simulink model "arduino"  (R2022a)
settings: Solver=VariableStepAuto  StartTime=0.0  StopTime=10.0  RelTol=1e-3
values from neighbouring files (symbols this model uses):
  R_L = 287    [ac_init.m]
libraries: eeGeneralControl x5, simulink x3, slpidlib x2, aerolibatmos2 x1
settings Model: Creator=vzink  LastModifiedBy=vzink

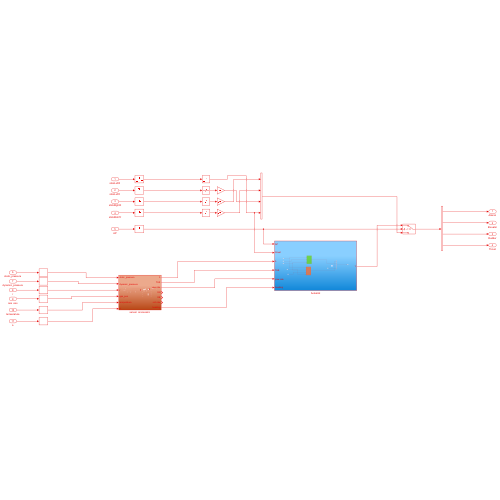
[thumbnail: Simulink's stored preview of the top-level diagram]
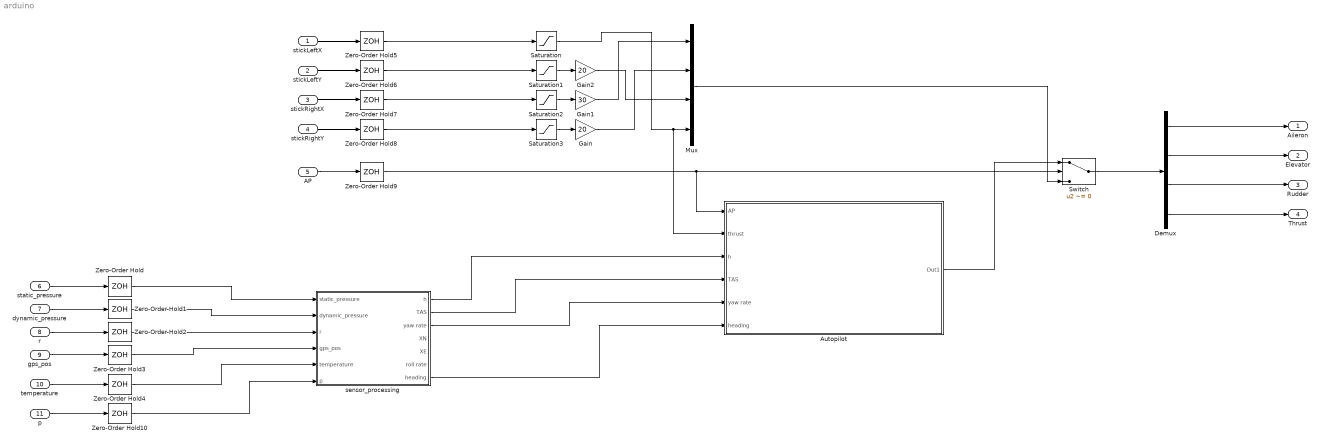
== system arduino ==
  stickLeftX : Inport
  stickLeftY : Inport  Port=2
  stickRightX : Inport  Port=3
  stickRightY : Inport  Port=4
  AP : Inport  Port=5
  static_pressure : Inport  Port=6
  dynamic_pressure : Inport  Port=7
  r : Inport  Port=8
  gps_pos : Inport  Port=9
  temperature : Inport  Port=10
  p : Inport  Port=11
  Autopilot : Subsystem
  Demux : Demux
  Gain : Gain  Gain=20
  Gain1 : Gain  Gain=30
  Gain2 : Gain  Gain=20
  Mux : Mux
  Saturation{,1..3} (4 alike) : Saturate  UpperLimit=1  LowerLimit=-1
  Switch : Switch  Criteria=u2 ~= 0  SaturateOnIntegerOverflow=off  InputSameDT=off
  Zero-Order Hold{,1..10} (11 alike) : ZeroOrderHold  SampleTime=0.01
  sensor_processing : Subsystem
  Aileron : Outport
  Elevator : Outport  Port=2
  Rudder : Outport  Port=3
  Thrust : Outport  Port=4
  wires:
  stickLeftX/1 -> Zero-Order Hold5/1
  stickLeftY/1 -> Zero-Order Hold6/1
  stickRightX/1 -> Zero-Order Hold7/1
  stickRightY/1 -> Zero-Order Hold8/1
  Saturation1/1 -> Gain2/1
  Saturation2/1 -> Gain1/1
  Saturation3/1 -> Gain/1
  Gain2/1 -> Mux/3
  Gain1/1 -> Mux/1
  Gain/1 -> Mux/2
  Saturation/1 -> Autopilot/2(thrust), Mux/4
  Mux/1 -> Switch/3
  Demux/1 -> Aileron/1
  Demux/2 -> Elevator/1
  Demux/3 -> Rudder/1
  Demux/4 -> Thrust/1
  Switch/1 -> Demux/1
  AP/1 -> Zero-Order Hold9/1
  static_pressure/1 -> Zero-Order Hold/1
  dynamic_pressure/1 -> Zero-Order Hold1/1
  r/1 -> Zero-Order Hold2/1
  gps_pos/1 -> Zero-Order Hold3/1
  temperature/1 -> Zero-Order Hold4/1
  sensor_processing/1(h) -> Autopilot/3(h)
  sensor_processing/2(TAS) -> Autopilot/4(TAS)
  sensor_processing/3(yaw rate) -> Autopilot/5(yaw rate)
  Zero-Order Hold/1 -> sensor_processing/1(static_pressure)
  Zero-Order Hold1/1 -> sensor_processing/2(dynamic_pressure)
  Zero-Order Hold2/1 -> sensor_processing/3(r)
  Zero-Order Hold3/1 -> sensor_processing/4(gps_pos)
  Zero-Order Hold4/1 -> sensor_processing/5(temperature)
  Zero-Order Hold5/1 -> Saturation/1
  Zero-Order Hold6/1 -> Saturation1/1
  Zero-Order Hold7/1 -> Saturation2/1
  Zero-Order Hold8/1 -> Saturation3/1
  Zero-Order Hold9/1 -> Autopilot/1(AP), Switch/2
  p/1 -> Zero-Order Hold10/1
  Zero-Order Hold10/1 -> sensor_processing/6(p)
  Autopilot/1(Out1) -> Switch/1
  sensor_processing/7(heading) -> Autopilot/6(heading)

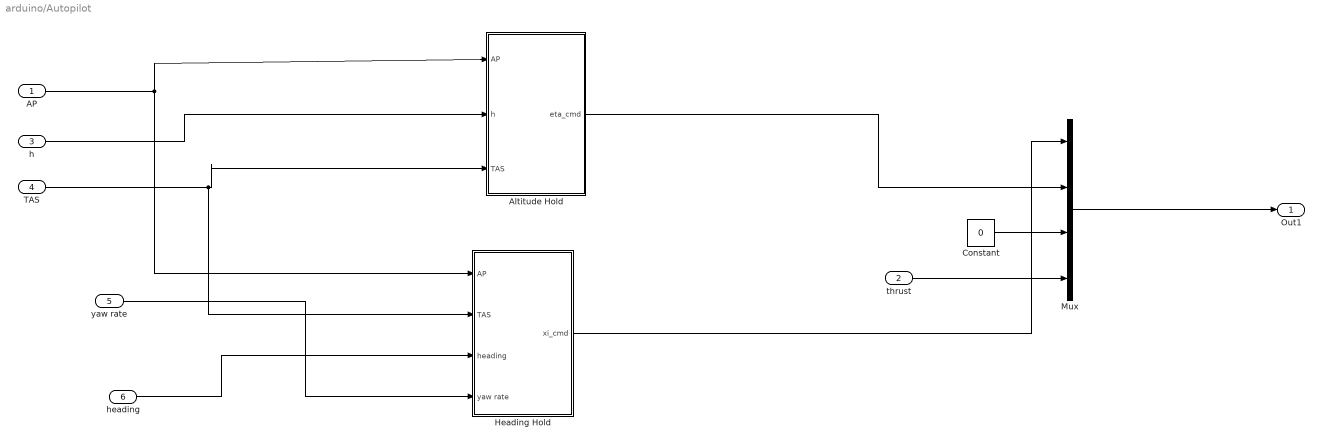
== system arduino/Autopilot ==
  AP : Inport
  thrust : Inport  Port=2
  h : Inport  Port=3
  TAS : Inport  Port=4
  yaw rate : Inport  Port=5
  heading : Inport  Port=6
  Altitude Hold : Subsystem
  Constant : Constant  Value=0
  Heading Hold : Subsystem
  Mux : Mux
  Out1 : Outport
  wires:
  Mux/1 -> Out1/1
  AP/1 -> Altitude Hold/1(AP), Heading Hold/1(AP)
  h/1 -> Altitude Hold/2(h)
  TAS/1 -> Heading Hold/2(TAS), Altitude Hold/3(TAS)
  Altitude Hold/1(eta_cmd) -> Mux/2
  thrust/1 -> Mux/4
  Constant/1 -> Mux/3
  Heading Hold/1(xi_cmd) -> Mux/1
  yaw rate/1 -> Heading Hold/4(yaw rate)
  heading/1 -> Heading Hold/3(heading)

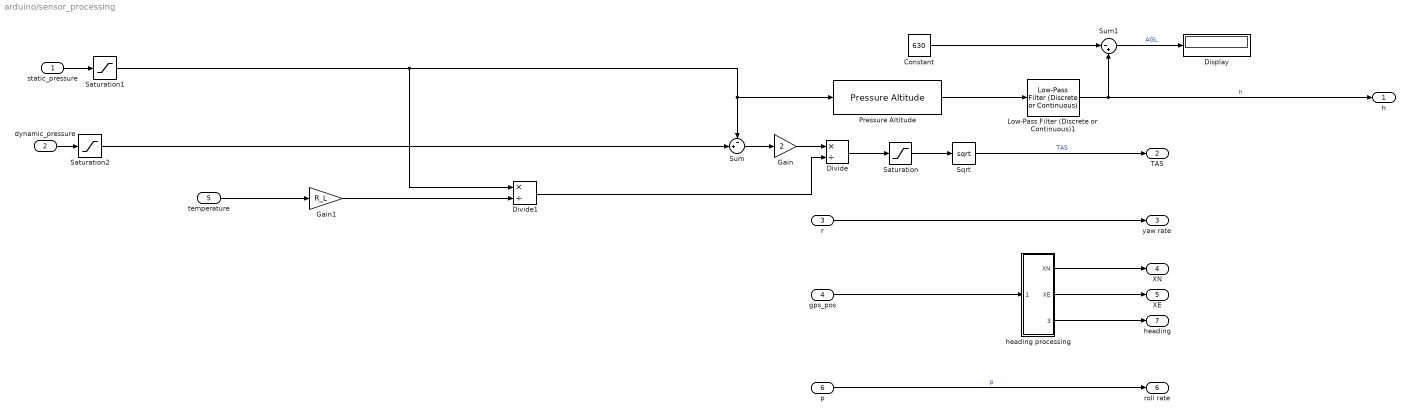
== system arduino/sensor_processing ==
  static_pressure : Inport
  dynamic_pressure : Inport  Port=2
  r : Inport  Port=3
  gps_pos : Inport  Port=4
  temperature : Inport  Port=5
  p : Inport  Port=6
  Constant : Constant  Value=630
  Display : Display
  Divide : Product  Inputs=*/
  Divide1 : Product  Inputs=*/
  Gain : Gain  Gain=2
  Gain1 : Gain  Gain=R_L
  Low-Pass Filter (Discrete or Continuous)1 : eeGeneralControl/Low-Pass Filter (Discrete or Continuous)  K=1  T=0.5  B=inf  A=-inf  init_option=Inherited from block input  x0=0  Ts=-1
  Pressure Altitude : aerolibatmos2/Pressure Altitude  units=Metric (MKS)  action=Warning
      settings: SourceProductBaseCode=AE
  Saturation : Saturate  UpperLimit=inf  LowerLimit=0
  Saturation1 : Saturate  UpperLimit=103000  LowerLimit=70000
  Saturation2 : Saturate  UpperLimit=103000  LowerLimit=70000
  Sqrt : Sqrt
  Sum : Sum  Inputs=-+|
  Sum1 : Sum  Inputs=|-+
  heading processing : Subsystem
  h : Outport
  TAS : Outport  Port=2
  yaw rate : Outport  Port=3
  XN : Outport  Port=4
  XE : Outport  Port=5
  roll rate : Outport  Port=6
  heading : Outport  Port=7
  wires:
  r/1 -> yaw rate/1
  static_pressure/1 -> Saturation1/1
  dynamic_pressure/1 -> Saturation2/1
  Sum/1 -> Gain/1
  Gain/1 -> Divide/1
  Divide/1 -> Saturation/1
  Sqrt/1 -> TAS/1  "TAS"
  Divide1/1 -> Divide/2
  Gain1/1 -> Divide1/2
  temperature/1 -> Gain1/1
  Saturation/1 -> Sqrt/1
  Pressure Altitude/1 -> Low-Pass Filter (Discrete or Continuous)1/1
  Constant/1 -> Sum1/1
  Sum1/1 -> Display/1  "AGL"
  Saturation1/1 -> Divide1/1, Pressure Altitude/1, Sum/1
  Saturation2/1 -> Sum/2
  Low-Pass Filter (Discrete or Continuous)1/1 -> h/1, Sum1/2  "h"
  p/1 -> roll rate/1  "p"
  gps_pos/1 -> heading processing/1(gps)
  heading processing/1(XN) -> XN/1
  heading processing/2(XE) -> XE/1
  heading processing/3(heading) -> heading/1

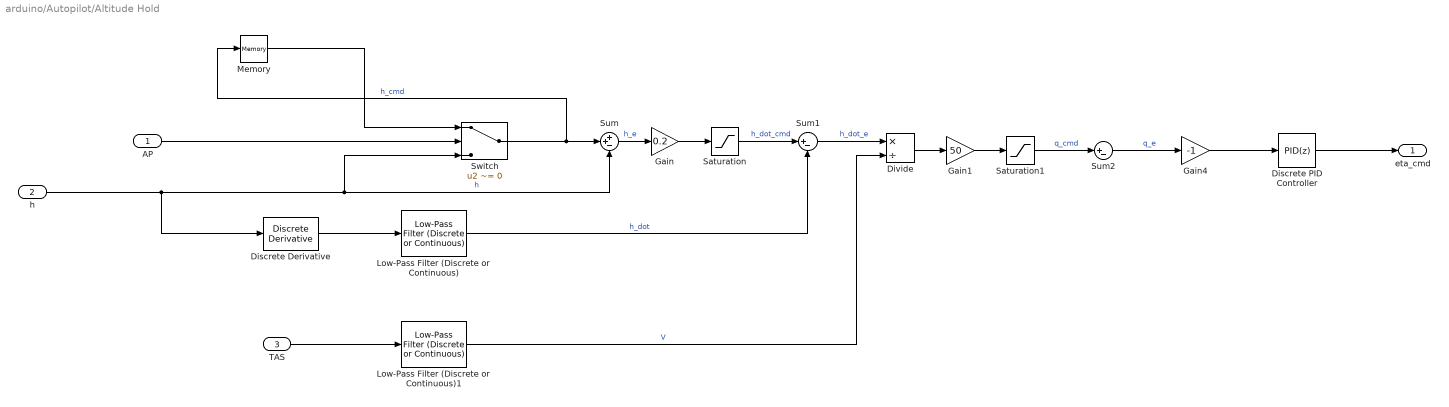
== system arduino/Autopilot/Altitude Hold ==
  AP : Inport
  h : Inport  Port=2
  TAS : Inport  Port=3
  Discrete Derivative : simulink/Discrete/Discrete Derivative  gainval=1.0  ICPrevScaledInput=730/0.01  OutMin=[]  OutMax=[]  OutDataType=fixdt(1, 16)  OutScaling=2^-10  DoSatur=off
  Discrete PID Controller : slpidlib/PID Controller  Controller=PID  Form=Parallel  TimeDomain=Discrete-time  UseExternalTs=off  SampleTime=-1  IntegratorMethod=Forward Euler  FilterMethod=Forward Euler  ControllerParametersSource=internal  P=2  I=0.05  UseKiTs=off  D=0  N=100  UseFilter=on  TunerSelectOption=Transfer Function Based (PID Tuner App)  InitialConditionSource=internal  InitialConditionForIntegrator=0  InitialConditionForFilter=0  DifferentiatorICPrevScaledInput=0  ExternalReset=none  TrackingMode=off  Kt=1  LimitOutput=off  SatLimitsSource=internal  UpperSaturationLimit=inf  LowerSaturationLimit=-inf  LinearizeAsGain=off  AntiWindupMode=none  Kb=1  POutMin=[]  POutMax=[]  IOutMin=[]  IOutMax=[]  DOutMin=[]  DOutMax=[]  NOutMin=[]  NOutMax=[]  SumOutMin=[]  SumOutMax=[]  SaturationOutMin=[]  SaturationOutMax=[]  PParamMin=[]  PParamMax=[]  IParamMin=[]  IParamMax=[]  DParamMin=[]  DParamMax=[]  NParamMin=[]  NParamMax=[]  KbParamMin=[]  KbParamMax=[]  KtParamMin=[]  KtParamMax=[]  KbOutMin=[]  KbOutMax=[]  KtOutMin=[]  KtOutMax=[]  IntegratorOutMin=[]  IntegratorOutMax=[]  FilterOutMin=[]  FilterOutMax=[]  SumI1OutMin=[]  SumI1OutMax=[]  SumI2OutMin=[]  SumI2OutMax=[]  SumI3OutMin=[]  SumI3OutMax=[]  SumI4OutMin=[]  SumI4OutMax=[]  SumDOutMin=[]  SumDOutMax=[]  DifferentiatorOutMin=[]  DifferentiatorOutMax=[]  FilterDiffOutCoefMin=[]  FilterDiffOutCoefMax=[]  ReciprocalOutMin=[]  ReciprocalOutMax=[]  SumDenOutMin=[]  SumDenOutMax=[]  SumNumOutMin=[]  SumNumOutMax=[]  DivideOutMin=[]  DivideOutMax=[]  UdiffTsProdOutMin=[]  UdiffTsProdOutMax=[]  NTsProdOutMin=[]  NTsProdOutMax=[]  UintegralTsProdOutMin=[]  UintegralTsProdOutMax=[]  UngainTsProdOutMin=[]  UngainTsProdOutMax=[]  IntegratorContinuousStateAttributes=''  IntegratorStateMustResolveToSignalObject=off  IntegratorRTWStateStorageClass=Auto  FilterContinuousStateAttributes=''  FilterStateMustResolveToSignalObject=off  FilterRTWStateStorageClass=Auto  ParallelPVariant=InternalParameters  IdealPVariant=Disabled  IVariant=InternalParameters  DVariant=InternalParameters  IntegratorVariant=Discrete  SatVariant=Disabled  AWVariant=Passthrough  PCopyVariant=Disabled  TRVariant=Disabled  FdbkBlocksVariant=Forward  IdealPFdbkVariant=Disabled  SatFdbkVariant=Disabled  DerivativeFilterVariant=ForwardEulerFilter  NVariant=InternalParameters  NCopyVariant=Disabled  FilterICVariant=InternalICsFilter  IntegratorICVariant=InternalICs  ExternalResetVariant=Disabled  TRSumVariant=Passthrough  SumFdbkVariant=Disabled  SumVariant=Sum_PID  TsampFilterVariant=InternalTs  TsampNgainVariant=Passthrough  TsampIntegralVariant=Passthrough  ExternalSaturationOutDataTypeStr=Inherit: Same as second input  aMode=0
  Divide : Product  Inputs=*/
  Gain : Gain  Gain=0.2
  Gain1 : Gain  Gain=50
  Gain4 : Gain  Gain=-1
  Low-Pass Filter (Discrete or Continuous) : eeGeneralControl/Low-Pass Filter (Discrete or Continuous)  K=1  T=1  B=inf  A=-inf  init_option=Inherited from block input  x0=0  Ts=-1
  Low-Pass Filter (Discrete or Continuous)1 : eeGeneralControl/Low-Pass Filter (Discrete or Continuous)  K=1  T=1  B=inf  A=-inf  init_option=Inherited from block input  x0=0  Ts=-1
  Memory : Memory  InheritSampleTime=on
  Saturation : Saturate  UpperLimit=1  LowerLimit=-1
  Saturation1 : Saturate  UpperLimit=10  LowerLimit=-10
  Sum : Sum  Inputs=++-
  Sum1 : Sum  Inputs=|+-
  Sum2 : Sum  Inputs=|+-
  Switch : Switch  Criteria=u2 ~= 0  SaturateOnIntegerOverflow=off  InputSameDT=off
  eta_cmd : Outport
  wires:
  Memory/1 -> Switch/1
  Switch/1 -> Memory/1, Sum/2  "h_cmd"
  AP/1 -> Switch/2
  Sum/1 -> Gain/1  "h_e"
  Gain/1 -> Saturation/1
  Saturation/1 -> Sum1/1  "h_dot_cmd"
  Discrete Derivative/1 -> Low-Pass Filter (Discrete or Continuous)/1
  h/1 -> Discrete Derivative/1, Sum/3, Switch/3  "h"
  Low-Pass Filter (Discrete or Continuous)/1 -> Sum1/2  "h_dot"
  TAS/1 -> Low-Pass Filter (Discrete or Continuous)1/1
  Low-Pass Filter (Discrete or Continuous)1/1 -> Divide/2  "V"
  Sum1/1 -> Divide/1  "h_dot_e"
  Divide/1 -> Gain1/1
  Gain1/1 -> Saturation1/1
  Sum2/1 -> Gain4/1  "q_e"
  Saturation1/1 -> Sum2/1  "q_cmd"
  Gain4/1 -> Discrete PID Controller/1
  Discrete PID Controller/1 -> eta_cmd/1

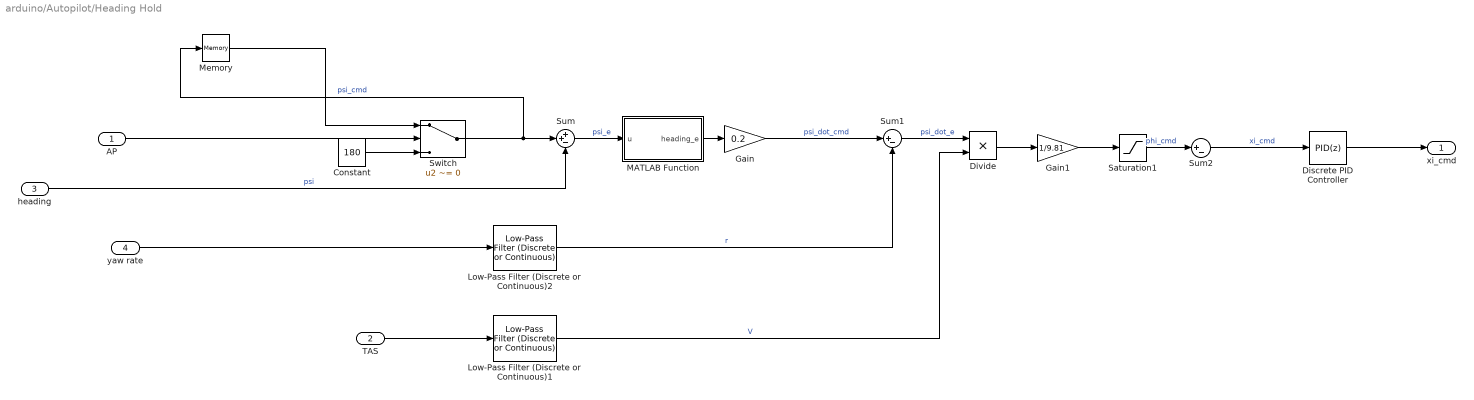
== system arduino/Autopilot/Heading Hold ==
  AP : Inport
  TAS : Inport  Port=2
  heading : Inport  Port=3
  yaw rate : Inport  Port=4
  Constant : Constant  Value=180
  Discrete PID Controller : slpidlib/PID Controller  Controller=PID  Form=Parallel  TimeDomain=Discrete-time  UseExternalTs=off  SampleTime=-1  IntegratorMethod=Forward Euler  FilterMethod=Forward Euler  ControllerParametersSource=internal  P=1  I=0  UseKiTs=off  D=0  N=100  UseFilter=on  TunerSelectOption=Transfer Function Based (PID Tuner App)  InitialConditionSource=internal  InitialConditionForIntegrator=0  InitialConditionForFilter=0  DifferentiatorICPrevScaledInput=0  ExternalReset=none  TrackingMode=off  Kt=1  LimitOutput=off  SatLimitsSource=internal  UpperSaturationLimit=inf  LowerSaturationLimit=-inf  LinearizeAsGain=off  AntiWindupMode=none  Kb=1  POutMin=[]  POutMax=[]  IOutMin=[]  IOutMax=[]  DOutMin=[]  DOutMax=[]  NOutMin=[]  NOutMax=[]  SumOutMin=[]  SumOutMax=[]  SaturationOutMin=[]  SaturationOutMax=[]  PParamMin=[]  PParamMax=[]  IParamMin=[]  IParamMax=[]  DParamMin=[]  DParamMax=[]  NParamMin=[]  NParamMax=[]  KbParamMin=[]  KbParamMax=[]  KtParamMin=[]  KtParamMax=[]  KbOutMin=[]  KbOutMax=[]  KtOutMin=[]  KtOutMax=[]  IntegratorOutMin=[]  IntegratorOutMax=[]  FilterOutMin=[]  FilterOutMax=[]  SumI1OutMin=[]  SumI1OutMax=[]  SumI2OutMin=[]  SumI2OutMax=[]  SumI3OutMin=[]  SumI3OutMax=[]  SumI4OutMin=[]  SumI4OutMax=[]  SumDOutMin=[]  SumDOutMax=[]  DifferentiatorOutMin=[]  DifferentiatorOutMax=[]  FilterDiffOutCoefMin=[]  FilterDiffOutCoefMax=[]  ReciprocalOutMin=[]  ReciprocalOutMax=[]  SumDenOutMin=[]  SumDenOutMax=[]  SumNumOutMin=[]  SumNumOutMax=[]  DivideOutMin=[]  DivideOutMax=[]  UdiffTsProdOutMin=[]  UdiffTsProdOutMax=[]  NTsProdOutMin=[]  NTsProdOutMax=[]  UintegralTsProdOutMin=[]  UintegralTsProdOutMax=[]  UngainTsProdOutMin=[]  UngainTsProdOutMax=[]  IntegratorContinuousStateAttributes=''  IntegratorStateMustResolveToSignalObject=off  IntegratorRTWStateStorageClass=Auto  FilterContinuousStateAttributes=''  FilterStateMustResolveToSignalObject=off  FilterRTWStateStorageClass=Auto  ParallelPVariant=InternalParameters  IdealPVariant=Disabled  IVariant=InternalParameters  DVariant=InternalParameters  IntegratorVariant=Discrete  SatVariant=Disabled  AWVariant=Passthrough  PCopyVariant=Disabled  TRVariant=Disabled  FdbkBlocksVariant=Forward  IdealPFdbkVariant=Disabled  SatFdbkVariant=Disabled  DerivativeFilterVariant=ForwardEulerFilter  NVariant=InternalParameters  NCopyVariant=Disabled  FilterICVariant=InternalICsFilter  IntegratorICVariant=InternalICs  ExternalResetVariant=Disabled  TRSumVariant=Passthrough  SumFdbkVariant=Disabled  SumVariant=Sum_PID  TsampFilterVariant=InternalTs  TsampNgainVariant=Passthrough  TsampIntegralVariant=Passthrough  ExternalSaturationOutDataTypeStr=Inherit: Same as second input  aMode=0
  Divide : Product
  Gain : Gain  Gain=0.2
  Gain1 : Gain  Gain=1/9.81
  Low-Pass Filter (Discrete or Continuous)1 : eeGeneralControl/Low-Pass Filter (Discrete or Continuous)  K=1  T=1  B=inf  A=-inf  init_option=Inherited from block input  x0=0  Ts=-1
  Low-Pass Filter (Discrete or Continuous)2 : eeGeneralControl/Low-Pass Filter (Discrete or Continuous)  K=1  T=0.001  B=inf  A=-inf  init_option=Inherited from block input  x0=0  Ts=-1
  MATLAB Function : MATLAB Function  TreatAsAtomicUnit=on
  Memory : Memory  InheritSampleTime=on
  Saturation1 : Saturate  UpperLimit=30  LowerLimit=-30
  Sum : Sum  Inputs=++-
  Sum1 : Sum  Inputs=|+-
  Sum2 : Sum  Inputs=|+-
  Switch : Switch  Criteria=u2 ~= 0  SaturateOnIntegerOverflow=off  InputSameDT=off
  xi_cmd : Outport
  wires:
  Discrete PID Controller/1 -> xi_cmd/1
  Saturation1/1 -> Sum2/1  "phi_cmd"
  Gain1/1 -> Saturation1/1
  Divide/1 -> Gain1/1
  Sum1/1 -> Divide/1  "psi_dot_e"
  Low-Pass Filter (Discrete or Continuous)1/1 -> Divide/2  "V"
  TAS/1 -> Low-Pass Filter (Discrete or Continuous)1/1
  heading/1 -> Sum/3  "psi"
  Gain/1 -> Sum1/1  "psi_dot_cmd"
  Sum/1 -> MATLAB Function/1(u)  "psi_e"
  AP/1 -> Switch/2
  Switch/1 -> Sum/2, Memory/1  "psi_cmd"
  Memory/1 -> Switch/1
  yaw rate/1 -> Low-Pass Filter (Discrete or Continuous)2/1
  Low-Pass Filter (Discrete or Continuous)2/1 -> Sum1/2  "r"
  MATLAB Function/1(heading_e) -> Gain/1
  Constant/1 -> Switch/3
  Sum2/1 -> Discrete PID Controller/1  "xi_cmd"

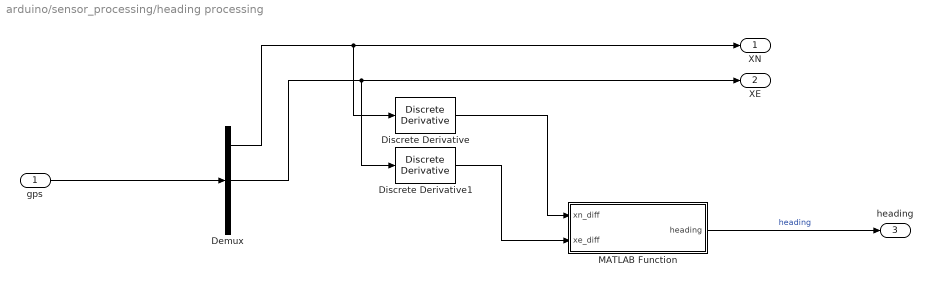
== system arduino/sensor_processing/heading processing ==
  gps : Inport
  Demux : Demux  Outputs=3
  Discrete Derivative : simulink/Discrete/Discrete Derivative  gainval=1.0  ICPrevScaledInput=0.0  OutMin=[]  OutMax=[]  OutDataType=fixdt(1, 16)  OutScaling=2^-10  DoSatur=off
  Discrete Derivative1 : simulink/Discrete/Discrete Derivative  gainval=1.0  ICPrevScaledInput=0.0  OutMin=[]  OutMax=[]  OutDataType=fixdt(1, 16)  OutScaling=2^-10  DoSatur=off
  MATLAB Function : MATLAB Function  TreatAsAtomicUnit=on
  XN : Outport
  XE : Outport  Port=2
  heading : Outport  Port=3
  wires:
  Demux/1 -> Discrete Derivative/1, XN/1
  Demux/2 -> Discrete Derivative1/1, XE/1
  gps/1 -> Demux/1
  Discrete Derivative/1 -> MATLAB Function/1(xn_diff)
  Discrete Derivative1/1 -> MATLAB Function/2(xe_diff)
  MATLAB Function/1(heading) -> heading/1  "heading"

== matlab function arduino/sensor_processing/heading processing/MATLAB Function ==
  data: xn_diff input; heading output; xe_diff input
function heading = fcn(xn_diff, xe_diff)

heading = mod(atan2d(xe_diff,xn_diff),360);

end

== matlab function arduino/Autopilot/Heading Hold/MATLAB Function ==
  data: u input; heading_e output
function heading_e = flip(u)
if u>180
    heading_e = -(360-u);
else
    heading_e = u;
end
end
